simulink model "HeadlessAttControllerVariableQuadDynamicsMdl"  (R2016b)
settings: Solver=FixedStepAuto  StartTime=0.0  StopTime=10  FixedStep=1/1000  RelTol=1e-3  EnableMultiTasking=on
undefined symbols (not defined in the file): Params, QuaternionControllerAtt
libraries: simulink x3
settings Model: Creator=Raj  LastModifiedBy=Hans
settings DataIOCC: LimitDataPoints=on  SaveFormat=Array
settings OptimizationCC: LifeSpan=inf
settings DebuggingCC: UnderspecifiedInitializationDetection=Classic  MergeDetectMultiDrivingBlocksExec=none  SolverPrmCheckMsg=warning  StateNameClashWarn=warning  SFUnexpectedBacktrackingDiag=warning  SFNoUnconditionalDefaultTransitionDiag=warning  SFExecutionAtInitializationDiag=none
settings HardwareCC: ProdBitPerPointer=32  ProdBitPerSizeT=32  ProdBitPerPtrDiffT=32  ProdLargestAtomicFloat=None  ProdIntDivRoundTo=Undefined  ProdEndianess=Unspecified  ProdWordSize=32  ProdHWDeviceType=32-bit Generic
settings ModelReferenceCC: PropagateSignalLabelsOutOfModel=off
settings GRTTargetCC: TargetLangStandard=C89/C90 (ANSI)  GeneratePreprocessorConditionals=Disable all
settings ConfigComp: CovMetricSettings=dw  CovHtmlReporting=on  CovSaveCumulativeToWorkspaceVar=on  CovSaveSingleToWorkspaceVar=on  CovExternalEMLEnable=off  CovSFcnEnable=off

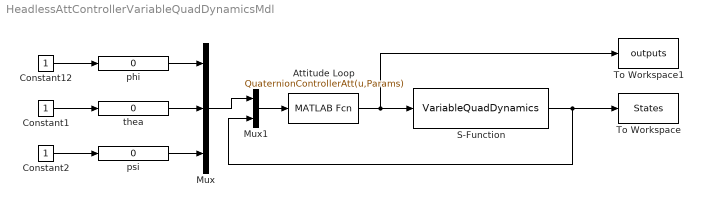
== system HeadlessAttControllerVariableQuadDynamicsMdl ==
  Attitude Loop : MATLABFcn  MATLABFcn=QuaternionControllerAtt(u,Params)  OutputDimensions=4
  Constant1 : Constant
  Constant12 : Constant
  Constant2 : Constant
  Mux : Mux  Inputs=3
  Mux1 : Mux  Inputs=2
  S-Function : S-Function  FunctionName=VariableQuadDynamics  Parameters=Params  SFunctionDeploymentMode=off  EnableBusSupport=off
  To Workspace : ToWorkspace  VariableName=States  SaveFormat=Timeseries  SampleTime=-1
  To Workspace1 : ToWorkspace  VariableName=outputs  SaveFormat=Timeseries  SampleTime=-1
  phi : simulink/Math Operations/Slider Gain  low=-20  gain=0  high=360
  psi : simulink/Math Operations/Slider Gain  low=-10  gain=0  high=10
  thea : simulink/Math Operations/Slider Gain  low=-20  gain=0  high=360
  wires:
  Constant12/1 -> phi/1
  Constant2/1 -> psi/1
  psi/1 -> Mux/3
  phi/1 -> Mux/1
  Attitude Loop/1 -> S-Function/1, To Workspace1/1
  Mux1/1 -> Attitude Loop/1
  Mux/1 -> Mux1/1
  S-Function/1 -> Mux1/2, To Workspace/1
  Constant1/1 -> thea/1
  thea/1 -> Mux/2
